simulink model "Electrical_System_2018b_obfs"  (R2019b)
settings: Solver=VariableStepAuto  StartTime=0.0  StopTime=5  RelTol=1e-3  AbsTol=1e-3  EnableMultiTasking=on
InitFcn:
  | Steady_State_Initialisation;
StopFcn:
  | %sscexplore(simlog);
  | %Logging
undefined symbols (not defined in the file): abrlhklxvp, aexgmhuedq, afmfmjnutg, afpphrjpnc, ahuxbyvruc, alarvljztt, amxnyqmnuw, aodrlwvqie, aolhmuplyq, aqpmguuqkg, auesgwirzl, aurophlnng, awamelrhru, ayfhvxflxn, azxkacuhqc, babszerikg, bawhdqanwq, bevoqecvei, bltjvqbchx, bmqsuewujl, bsmyqjfgnf, btvjbsmnve, bywgxqeadw, bziaduxaer, bzmcmdqocb, bzsvyvetat, ccsjnrbsih, cdvenygxwh, cedkrnslhx, cjheorclzs, cjrdshrtqx, ckhavyhcza, ckxewznhlz, cmrcgyiplk, conenicnws, cqkejbgjnn, csfnuwymhe, cunupkhwbh, cwzfvzuxxh, dcadmadufn, dcfponivnv, ddtrqjrhjn, dfhoxvkqas, dfrhtcwpne, dfvomcagjv, djijwylxea, dnmeqksrrm, dnzewbdkaa, dsqcykyxav, dtswwlttmm, ecumpidjtv, edegaywrct, ejjjsmnejc, eknqnehjdz, emvdetzouf, esxbqkbahr, etnkkbreiq, eunoiiiirw, ewewcuedir, fatkfxdhtc ... (+386)
libraries: fl_lib x802, ee_lib x362, fl_ps_legacy_lib x160, nesl_utility x85
(part 17 of 26)

== system Electrical_System_2018b_obfs/Redacted_1221/Redacted_7996/Redacted_7418/Redacted_4377/Redacted_6082/Redacted_1658 ==
  Redacted_1005 : fl_lib/Electrical/Electrical Elements/Switch  R_closed=ejlyeridsw Ohm  G_open=efsydslasd 1/Ohm  Threshold=qludltxvzj  i_specify=off  i_priority=None  i=qtqqggocjg A  i_nominal_specify=off  i_nominal_unit=A  i_nominal_value=irfgdwsyws  v_specify=off  v_priority=None  v=nrsfaplzum V  v_nominal_specify=off  v_nominal_unit=V  v_nominal_value=ffnnoojtnr
      settings: SourceProductName=Simscape
  Redacted_1354 : ee_lib/Passive/Thermal/Thermal Resistor  R=qdgpqkdjpo K/W  T_specify=off  T_priority=None  T=mtinxqvpod K  T_nominal_specify=off  T_nominal_unit=K  T_nominal_value=nyetipzdbd  Q_specify=off  Q_priority=None  Q=zeibppilau W  Q_nominal_specify=off  Q_nominal_unit=W  Q_nominal_value=ovthkmdajp
      settings: SourceProductName=Simscape Electrical  SourceProductBaseCode=PS  InternalSimscapePortConfiguration="{\"Bottom\":[],\"Left\":[{\"id\":\"A\",\"label\":\"A\",\"type\":\"foundation.thermal.thermal\"}],\"Right\":[{\"id\":\"B\",\"label\":\"B\",\"type\":\"foundation.thermal.thermal\"}],\"Top\":[]}"
  Redacted_3286 : ee_lib/Semiconductors & Converters/Diode  ModelType=qyiuharngl  Vf=uavesysmzd V  Ron=izxucsnofw Ohm  Goff=hxvsqjqvfr S  prmExp=jwlbdrgdyn  I12=fhtaelyvur A  V12=pntclgauty V  IS=xlgdpvdion A  ec=lsuwwyvoaz  I1=xioaihhcoe A  V1=prlupfwjwk V  RS=grfujeuioo Ohm  Tmeas=mmahtgxtlp degC  N_series=bdqkkbdoww  N_parallel=bdgudnfeam  Rz=vsyxoldpzj Ohm  BV=rczxpthhgf V  C_param=tlcavagjol  CJ=ssqnkrbywq pF  CJ0=wrromkkilg pF  VJ=faazhshxub V  Mgrad=ldrovslsoh  Vvec=vtbaecghrb V  Cvec=rijvdbsbjz pF  FC=ouvrtbvulr  Q_param=rrrehddltc  iRM=fyquguupcf A  iF=ikkfryheqp A  didt=scbuuymmti A/us  trr_factor=vwdzzjgtdl  trr=zktlrrknks ns  Qrr=utuviybabn s*uA  TT=jcgggencbc ns  tau=ssflxvsiut ns  T_param=nblvkicsaj  IS_T2=hpuqfgybtl A  I1_T2=atejcpbsmg A  V1_T2=txapzmzmbr V  Tmeas2=hogrcmodsn degC  EG_param=fwyzdxmfgf  EG=zfrilvllus eV  XTI_param=gxndnzccej  XTI=zngcdbbpek  dBVdT=ultmrnqodj V/K  Tdevice=cvuddcjgoa degC  i_specify=off  i_priority=None  i=xckzxtcuri A  i_nominal_specify=off  i_nominal_unit=A  i_nominal_value=mfjascwvwx  v_specify=off  v_priority=None  v=oytsestkkt V  v_nominal_specify=off  v_nominal_unit=V  v_nominal_value=rbtpehkrox  i_capacitor_specify=off  i_capacitor_priority=None  i_capacitor=lydrbpwfwm A  i_capacitor_nominal_specify=off  i_capacitor_nominal_unit=A  i_capacitor_nominal_value=gsonjyrsiu  v_capacitor_specify=off  v_capacitor_priority=None  v_capacitor=tlqtmxeebh V  v_capacitor_nominal_specify=off  v_capacitor_nominal_unit=V  v_capacitor_nominal_value=ixflknqnnv  power_dissipated_specify=off  power_dissipated_priority=None  power_dissipated=vhmskoronr W  power_dissipated_nominal_specify=off  power_dissipated_nominal_unit=W  power_dissipated_nominal_value=rqgtxqlwdp  thermal_network_parameterization=xkaopcnmoj  Rth=skumtgliel K/W  Rth_Foster=widqwnvljq K/W  thermal_mass_parameterization=ihdtigkqdr  thermal_mass=fxsrzmeque J/K  thermal_mass_Foster=cbmthsfafj J/K  thermal_time_constant=pmaqruvvqr s  thermal_time_constant_Foster=pxvwqyklyc s  thermal_mass_initial_temperatures=qerohrajht degC
      settings: SourceProductName=Simscape Electrical  InternalSimscapePortConfiguration="{\"Bottom\":[],\"Left\":[{\"id\":\"p\",\"label\":\"\",\"type\":\"foundation.electrical.electrical\"},{\"id\":\"H\",\"label\":\"H\",\"type\":\"foundation.thermal.thermal\"}],\"Right\":[{\"id\":\"n\",\"label\":\"\",\"type\":\"foundation.electrical.electrical\"}],\"Top\":[]}"
  Redacted_3861 : ee_lib/Semiconductors & Converters/Diode  ModelType=fxgsrmkiul  Vf=nwkiuphnod V  Ron=ytonkdenqd Ohm  Goff=vvxokjkhhi S  prmExp=rjijseurnu  I12=plnpdpppsb A  V12=clscpnwkyn V  IS=fgyrvtcpjw A  ec=myarsmgyax  I1=zaiuznwqub A  V1=urqjkvkqaz V  RS=atpbcqwqrk Ohm  Tmeas=avxaumhyvi degC  N_series=bdgfkyrlsu  N_parallel=cgmwatvtyk  Rz=jwremjkbfv Ohm  BV=kmqlppxuzg V  C_param=vvtbjwiqjw  CJ=dvukuyjagk pF  CJ0=ajovvjufex pF  VJ=lqxioxyjxp V  Mgrad=ugprrqpcng  Vvec=aycruakske V  Cvec=grqlqlzqyb pF  FC=xafzerxcin  Q_param=vnlbkyokpw  iRM=myuopxdhnp A  iF=wopzcdppvb A  didt=yoejpqomll A/us  trr_factor=vnzcsazbfp  trr=flnrjlmhdl ns  Qrr=abhmmrvgxl s*uA  TT=gfztyjvgqq ns  tau=oustnvpcaz ns  T_param=aznyhdnxgk  IS_T2=boxomshjpr A  I1_T2=imlgomczsp A  V1_T2=bhyftvbhbd V  Tmeas2=bhksuazwhb degC  EG_param=asaybnfknm  EG=gsrzwalape eV  XTI_param=duwkdllyki  XTI=aszcjfwkon  dBVdT=xhavbsykud V/K  Tdevice=nfydvwwomt degC  i_specify=off  i_priority=None  i=hibpeusmqj A  i_nominal_specify=off  i_nominal_unit=A  i_nominal_value=dgpnvsgdwn  v_specify=off  v_priority=None  v=xzghpqhkll V  v_nominal_specify=off  v_nominal_unit=V  v_nominal_value=aqwbnuvuma  i_capacitor_specify=off  i_capacitor_priority=None  i_capacitor=dbdawzejgx A  i_capacitor_nominal_specify=off  i_capacitor_nominal_unit=A  i_capacitor_nominal_value=skfhqqsyjv  v_capacitor_specify=off  v_capacitor_priority=None  v_capacitor=kngohrnxjb V  v_capacitor_nominal_specify=off  v_capacitor_nominal_unit=V  v_capacitor_nominal_value=knpvixzgdi  power_dissipated_specify=off  power_dissipated_priority=None  power_dissipated=zhfsmmbryx W  power_dissipated_nominal_specify=off  power_dissipated_nominal_unit=W  power_dissipated_nominal_value=oxbqwsyfdo  thermal_network_parameterization=gluxlhswsh  Rth=wkzzkloygz K/W  Rth_Foster=lchzecrkjz K/W  thermal_mass_parameterization=gwvmgktbjo  thermal_mass=rmhlykpfbd J/K  thermal_mass_Foster=ahdrbmndbt J/K  thermal_time_constant=geccsojpnx s  thermal_time_constant_Foster=oeduphnpru s  thermal_mass_initial_temperatures=wnupirfodr degC
      settings: SourceProductName=Simscape Electrical  InternalSimscapePortConfiguration="{\"Bottom\":[],\"Left\":[{\"id\":\"p\",\"label\":\"\",\"type\":\"foundation.electrical.electrical\"},{\"id\":\"H\",\"label\":\"H\",\"type\":\"foundation.thermal.thermal\"}],\"Right\":[{\"id\":\"n\",\"label\":\"\",\"type\":\"foundation.electrical.electrical\"}],\"Top\":[]}"
  Redacted_5977 : fl_lib/Electrical/Electrical Elements/Switch  R_closed=cjwmmdrupk Ohm  G_open=qstxdugiyk 1/Ohm  Threshold=kztcpnpmvs  i_specify=off  i_priority=None  i=lmxbtdndwg A  i_nominal_specify=off  i_nominal_unit=A  i_nominal_value=qyeufjvfiw  v_specify=off  v_priority=None  v=gastazzonl V  v_nominal_specify=off  v_nominal_unit=V  v_nominal_value=mjiwwishzy
      settings: SourceProductName=Simscape
  Redacted_6041 : ee_lib/Passive/Thermal/Thermal Resistor  R=xbcnqysxek K/W  T_specify=off  T_priority=None  T=bzsvyvetat K  T_nominal_specify=off  T_nominal_unit=K  T_nominal_value=ewqiuajrkb  Q_specify=off  Q_priority=None  Q=jhzrvwpmgk W  Q_nominal_specify=off  Q_nominal_unit=W  Q_nominal_value=tohlmuixqc
      settings: SourceProductName=Simscape Electrical  SourceProductBaseCode=PS  InternalSimscapePortConfiguration="{\"Bottom\":[],\"Left\":[{\"id\":\"A\",\"label\":\"A\",\"type\":\"foundation.thermal.thermal\"}],\"Right\":[{\"id\":\"B\",\"label\":\"B\",\"type\":\"foundation.thermal.thermal\"}],\"Top\":[]}"
  Redacted_7612 : ee_lib/Passive/Thermal/Thermal Resistor  R=ogtgsqkykv K/W  T_specify=off  T_priority=None  T=welbpoxbdd K  T_nominal_specify=off  T_nominal_unit=K  T_nominal_value=owcjlhxdxh  Q_specify=off  Q_priority=None  Q=jawtmfuqev W  Q_nominal_specify=off  Q_nominal_unit=W  Q_nominal_value=amvswbkqpm
      settings: SourceProductName=Simscape Electrical  SourceProductBaseCode=PS  InternalSimscapePortConfiguration="{\"Bottom\":[],\"Left\":[{\"id\":\"A\",\"label\":\"A\",\"type\":\"foundation.thermal.thermal\"}],\"Right\":[{\"id\":\"B\",\"label\":\"B\",\"type\":\"foundation.thermal.thermal\"}],\"Top\":[]}"
  Redacted_4312 : PMIOPort  Side=Left
  Redacted_7440 : PMIOPort  Port=2  Side=Left
  Redacted_7574 : PMIOPort  Port=3  Side=Right
  Redacted_5998 : PMIOPort  Port=4  Side=Right
  Redacted_5346 : PMIOPort  Port=5  Side=Left
  Redacted_698 : PMIOPort  Port=6  Side=Right
  connections:
  Redacted_3861/LConn2 -- Redacted_7612/LConn1
  Redacted_6041/RConn1 -- Redacted_5346/RConn1
  Redacted_5998/RConn1 -- Redacted_5977/RConn2
  Redacted_1005/RConn1 -- Redacted_5977/RConn1 -- Redacted_698/RConn1
  Redacted_1354/RConn1 -- Redacted_6041/LConn1 -- Redacted_7612/RConn1
  Redacted_4312/RConn1 -- Redacted_3286/RConn1
  Redacted_3286/LConn1 -- Redacted_1005/LConn1
  Redacted_7574/RConn1 -- Redacted_1005/RConn2
  Redacted_3286/LConn2 -- Redacted_1354/LConn1
  Redacted_3861/RConn1 -- Redacted_5977/LConn1
  Redacted_3861/LConn1 -- Redacted_7440/RConn1

== system Electrical_System_2018b_obfs/Redacted_1221/Redacted_7996/Redacted_7418/Redacted_4377/Redacted_6082/Redacted_1843 ==
  Neutral_Negative : Subsystem  VariantControl=Variant1
  Positive_Neutral : Subsystem  VariantControl=Variant3
  Redacted_8971 : Subsystem  VariantControl=Variant2
  Redacted_2601 : PMIOPort  Side=Left
  Redacted_5367 : PMIOPort  Port=2  Side=Left
  Redacted_1109 : PMIOPort  Port=3  Side=Left
  Redacted_4235 : PMIOPort  Port=4  Side=Right
  Redacted_9086 : PMIOPort  Port=5  Side=Right

== system Electrical_System_2018b_obfs/Redacted_1221/Redacted_7996/Redacted_7418/Redacted_4377/Redacted_6082/Redacted_1901 ==
  Redacted_1229 : ee_lib/Passive/Thermal/Thermal Resistor  R=hfneeleggr K/W  T_specify=off  T_priority=None  T=dnmeqksrrm K  T_nominal_specify=off  T_nominal_unit=K  T_nominal_value=uhclxpopbh  Q_specify=off  Q_priority=None  Q=nyzppyukeu W  Q_nominal_specify=off  Q_nominal_unit=W  Q_nominal_value=mrympoiojz
      settings: SourceProductName=Simscape Electrical  SourceProductBaseCode=PS  InternalSimscapePortConfiguration="{\"Bottom\":[],\"Left\":[{\"id\":\"A\",\"label\":\"A\",\"type\":\"foundation.thermal.thermal\"}],\"Right\":[{\"id\":\"B\",\"label\":\"B\",\"type\":\"foundation.thermal.thermal\"}],\"Top\":[]}"
  Redacted_1317 : ee_lib/Passive/Thermal/Thermal Resistor  R=ddtrqjrhjn K/W  T_specify=off  T_priority=None  T=myvnfneauu K  T_nominal_specify=off  T_nominal_unit=K  T_nominal_value=vndthaumwj  Q_specify=off  Q_priority=None  Q=jvrrmptdue W  Q_nominal_specify=off  Q_nominal_unit=W  Q_nominal_value=zyzovxzrox
      settings: SourceProductName=Simscape Electrical  SourceProductBaseCode=PS  InternalSimscapePortConfiguration="{\"Bottom\":[],\"Left\":[{\"id\":\"A\",\"label\":\"A\",\"type\":\"foundation.thermal.thermal\"}],\"Right\":[{\"id\":\"B\",\"label\":\"B\",\"type\":\"foundation.thermal.thermal\"}],\"Top\":[]}"
  Redacted_2918 : ee_lib/Semiconductors & Converters/Diode  ModelType=tboxenabfk  Vf=ysocghjvnj V  Ron=igyyqbbazt Ohm  Goff=wrcmatehqh S  prmExp=umofwxphaz  I12=boewnunols A  V12=agfxygazzy V  IS=yxpwlphqya A  ec=ezskytlukg  I1=hfmdeevxjm A  V1=lbjfenfgli V  RS=crmaftxtdn Ohm  Tmeas=rzhxrfhrws degC  N_series=qhotvmyapg  N_parallel=dcamtsthwp  Rz=qwnnbscosu Ohm  BV=bgsuezylxr V  C_param=jefhggiqkq  CJ=nrftpgzbwn pF  CJ0=vpkmzxlujx pF  VJ=nqopqysaak V  Mgrad=jnpgifqefs  Vvec=cniqwxpvbi V  Cvec=plwpepcsqe pF  FC=gzewllqrkw  Q_param=xlnrldobms  iRM=ytqzliqbll A  iF=svsqnejsfr A  didt=lrnrbryckm A/us  trr_factor=qpcgqhjpel  trr=emvijkzjdz ns  Qrr=ykzfmghaqw s*uA  TT=cegrsucons ns  tau=hhbhhwwsxm ns  T_param=jxhekmoycn  IS_T2=cnunlqxwqa A  I1_T2=tqdiqvzzvb A  V1_T2=ukgedxicts V  Tmeas2=ypzgidmcky degC  EG_param=ahptxqtjkj  EG=pprjzflisz eV  XTI_param=luwukgfqqn  XTI=bnvhtyteod  dBVdT=loswkuonel V/K  Tdevice=ctewjlisga degC  i_specify=off  i_priority=None  i=kufuhybcxo A  i_nominal_specify=off  i_nominal_unit=A  i_nominal_value=fnodmzekrv  v_specify=off  v_priority=None  v=bvjjoninjh V  v_nominal_specify=off  v_nominal_unit=V  v_nominal_value=wmrqkzdvam  i_capacitor_specify=off  i_capacitor_priority=None  i_capacitor=sawezjxpgh A  i_capacitor_nominal_specify=off  i_capacitor_nominal_unit=A  i_capacitor_nominal_value=dzrakfqruq  v_capacitor_specify=off  v_capacitor_priority=None  v_capacitor=ckefveljbv V  v_capacitor_nominal_specify=off  v_capacitor_nominal_unit=V  v_capacitor_nominal_value=zlbmprnqfe  power_dissipated_specify=off  power_dissipated_priority=None  power_dissipated=npelzyxkbr W  power_dissipated_nominal_specify=off  power_dissipated_nominal_unit=W  power_dissipated_nominal_value=xyqqsiyxsx  thermal_network_parameterization=cmpqaimztb  Rth=fyfjdoegdn K/W  Rth_Foster=ouazsjqzqc K/W  thermal_mass_parameterization=uskugrezwe  thermal_mass=kfppvbxohl J/K  thermal_mass_Foster=iohubghcog J/K  thermal_time_constant=tbegstwujr s  thermal_time_constant_Foster=kbaqkpxwop s  thermal_mass_initial_temperatures=tmxmgoawom degC
      settings: SourceProductName=Simscape Electrical  InternalSimscapePortConfiguration="{\"Bottom\":[],\"Left\":[{\"id\":\"p\",\"label\":\"\",\"type\":\"foundation.electrical.electrical\"},{\"id\":\"H\",\"label\":\"H\",\"type\":\"foundation.thermal.thermal\"}],\"Right\":[{\"id\":\"n\",\"label\":\"\",\"type\":\"foundation.electrical.electrical\"}],\"Top\":[]}"
  Redacted_3887 : ee_lib/Semiconductors & Converters/Diode  ModelType=kgpqvwzuvf  Vf=pusmgjlfhw V  Ron=zdvhkofkio Ohm  Goff=rrsomwrhky S  prmExp=puvexjufpm  I12=tlbhkktqov A  V12=jgzzzcxugv V  IS=pqeeblyemi A  ec=yagdawcefa  I1=baiumjodsv A  V1=kvrziecayr V  RS=emddjdnqya Ohm  Tmeas=kukopsdiuw degC  N_series=rabuyhqlar  N_parallel=fzdlculjid  Rz=oyqbhoxixc Ohm  BV=powcerqowi V  C_param=aeoqkmsqgo  CJ=omumwwbzoq pF  CJ0=sznaxolwxw pF  VJ=kdgpnhjdki V  Mgrad=owoxwkiptx  Vvec=yphehuqnex V  Cvec=yioiudmgas pF  FC=diwfpfnlom  Q_param=cswgmtympe  iRM=nsikknuycn A  iF=udnoipznau A  didt=omhhheqqis A/us  trr_factor=kiajvubcqx  trr=eifapbzssj ns  Qrr=igpekaohrl s*uA  TT=jucdrpilud ns  tau=lahsbpxgyi ns  T_param=vnthpegzri  IS_T2=edtnoyclnw A  I1_T2=emvajrspsy A  V1_T2=nghezzebkw V  Tmeas2=etfqwqeleu degC  EG_param=fmhucqmugz  EG=ytvyyycxld eV  XTI_param=kxpyactpjk  XTI=ijcctumawz  dBVdT=mveoqdoxea V/K  Tdevice=rasndouawu degC  i_specify=off  i_priority=None  i=middmtxema A  i_nominal_specify=off  i_nominal_unit=A  i_nominal_value=ulcnzrhotg  v_specify=off  v_priority=None  v=cirgoxespi V  v_nominal_specify=off  v_nominal_unit=V  v_nominal_value=dnkswukuqy  i_capacitor_specify=off  i_capacitor_priority=None  i_capacitor=uvmqwudjqx A  i_capacitor_nominal_specify=off  i_capacitor_nominal_unit=A  i_capacitor_nominal_value=tjhsaljlzi  v_capacitor_specify=off  v_capacitor_priority=None  v_capacitor=gtauwsvkmg V  v_capacitor_nominal_specify=off  v_capacitor_nominal_unit=V  v_capacitor_nominal_value=yrtxkgmrjc  power_dissipated_specify=off  power_dissipated_priority=None  power_dissipated=gejrmthogs W  power_dissipated_nominal_specify=off  power_dissipated_nominal_unit=W  power_dissipated_nominal_value=fnkdipvfax  thermal_network_parameterization=brstcitzoq  Rth=qauyoickxf K/W  Rth_Foster=pcmfvqnjph K/W  thermal_mass_parameterization=csstahwskj  thermal_mass=uinbpeizom J/K  thermal_mass_Foster=udgsofajzw J/K  thermal_time_constant=fbszgisaxv s  thermal_time_constant_Foster=qzpyvzuxkn s  thermal_mass_initial_temperatures=tcrrrnbkcb degC
      settings: SourceProductName=Simscape Electrical  InternalSimscapePortConfiguration="{\"Bottom\":[],\"Left\":[{\"id\":\"p\",\"label\":\"\",\"type\":\"foundation.electrical.electrical\"},{\"id\":\"H\",\"label\":\"H\",\"type\":\"foundation.thermal.thermal\"}],\"Right\":[{\"id\":\"n\",\"label\":\"\",\"type\":\"foundation.electrical.electrical\"}],\"Top\":[]}"
  Redacted_5062 : fl_lib/Electrical/Electrical Elements/Switch  R_closed=ajgjjzldor Ohm  G_open=aanuvbeift 1/Ohm  Threshold=fyvpcwnmem  i_specify=off  i_priority=None  i=farnwkyrka A  i_nominal_specify=off  i_nominal_unit=A  i_nominal_value=uzlteuglkb  v_specify=off  v_priority=None  v=tekycmpguo V  v_nominal_specify=off  v_nominal_unit=V  v_nominal_value=hyrhbabztl
      settings: SourceProductName=Simscape
  Redacted_6145 : fl_lib/Electrical/Electrical Elements/Switch  R_closed=wzxtffzhqk Ohm  G_open=ttmifnbefi 1/Ohm  Threshold=zzdsjwvyov  i_specify=off  i_priority=None  i=wibaukydmt A  i_nominal_specify=off  i_nominal_unit=A  i_nominal_value=shaiddzzkm  v_specify=off  v_priority=None  v=adhjlkibew V  v_nominal_specify=off  v_nominal_unit=V  v_nominal_value=ctlxurrbzu
      settings: SourceProductName=Simscape
  Redacted_8303 : ee_lib/Passive/Thermal/Thermal Resistor  R=dcadmadufn K/W  T_specify=off  T_priority=None  T=kapvbwdbts K  T_nominal_specify=off  T_nominal_unit=K  T_nominal_value=ghgowxtkgp  Q_specify=off  Q_priority=None  Q=amzvaiirbc W  Q_nominal_specify=off  Q_nominal_unit=W  Q_nominal_value=ptxjogujxs
      settings: SourceProductName=Simscape Electrical  SourceProductBaseCode=PS  InternalSimscapePortConfiguration="{\"Bottom\":[],\"Left\":[{\"id\":\"A\",\"label\":\"A\",\"type\":\"foundation.thermal.thermal\"}],\"Right\":[{\"id\":\"B\",\"label\":\"B\",\"type\":\"foundation.thermal.thermal\"}],\"Top\":[]}"
  Redacted_8116 : PMIOPort  Side=Left
  Redacted_9290 : PMIOPort  Port=2  Side=Left
  Redacted_6411 : PMIOPort  Port=3  Side=Right
  Redacted_9481 : PMIOPort  Port=4  Side=Right
  Redacted_1243 : PMIOPort  Port=5  Side=Left
  Redacted_5181 : PMIOPort  Port=6  Side=Right
  connections:
  Redacted_3887/LConn1 -- Redacted_9290/RConn1
  Redacted_3887/RConn1 -- Redacted_6145/LConn1
  Redacted_2918/LConn2 -- Redacted_1229/LConn1
  Redacted_6411/RConn1 -- Redacted_5062/RConn2
  Redacted_2918/LConn1 -- Redacted_5062/LConn1
  Redacted_8116/RConn1 -- Redacted_2918/RConn1
  Redacted_1317/RConn1 -- Redacted_8303/LConn1 -- Redacted_1229/RConn1
  Redacted_5181/RConn1 -- Redacted_6145/RConn1 -- Redacted_5062/RConn1
  Redacted_9481/RConn1 -- Redacted_6145/RConn2
  Redacted_8303/RConn1 -- Redacted_1243/RConn1
  Redacted_3887/LConn2 -- Redacted_1317/LConn1

== system Electrical_System_2018b_obfs/Redacted_1221/Redacted_7996/Redacted_7418/Redacted_4377/Redacted_6082/Redacted_2005 ==
  Neutral_Negative : Subsystem  VariantControl=Variant1
  Positive_Neutral : Subsystem  VariantControl=Variant3
  Redacted_335 : Subsystem  VariantControl=Variant2
  Redacted_8266 : PMIOPort  Side=Left
  Redacted_1423 : PMIOPort  Port=2  Side=Left
  Redacted_7633 : PMIOPort  Port=3  Side=Left
  Redacted_8552 : PMIOPort  Port=4  Side=Right
  Redacted_2441 : PMIOPort  Port=5  Side=Right

== system Electrical_System_2018b_obfs/Redacted_1221/Redacted_7996/Redacted_7418/Redacted_4377/Redacted_6082/Redacted_2122 ==
  Neutral_Negative : Subsystem  VariantControl=Variant1
  Positive_Neutral : Subsystem  VariantControl=Variant3
  Redacted_1391 : Subsystem  VariantControl=Variant2
  Redacted_659 : PMIOPort  Side=Left
  Redacted_1619 : PMIOPort  Port=2  Side=Left
  Redacted_5171 : PMIOPort  Port=3  Side=Left
  Redacted_2219 : PMIOPort  Port=4  Side=Right
  Redacted_5591 : PMIOPort  Port=5  Side=Right

== system Electrical_System_2018b_obfs/Redacted_1221/Redacted_7996/Redacted_7418/Redacted_4377/Redacted_6082/Redacted_2183 ==
  Redacted_1396 : fl_lib/Electrical/Electrical Elements/Switch  R_closed=wmcpxqyfeh Ohm  G_open=ordboroxst 1/Ohm  Threshold=puyanqdwrl  i_specify=off  i_priority=None  i=bnajmanprt A  i_nominal_specify=off  i_nominal_unit=A  i_nominal_value=rlbcudmlql  v_specify=off  v_priority=None  v=cqbyhwtmeu V  v_nominal_specify=off  v_nominal_unit=V  v_nominal_value=ssehunbzon
      settings: SourceProductName=Simscape
  Redacted_3366 : ee_lib/Passive/Thermal/Thermal Resistor  R=bawhdqanwq K/W  T_specify=off  T_priority=None  T=nptyawlpaq K  T_nominal_specify=off  T_nominal_unit=K  T_nominal_value=finlbxanjw  Q_specify=off  Q_priority=None  Q=alilpavgri W  Q_nominal_specify=off  Q_nominal_unit=W  Q_nominal_value=wneqapuicx
      settings: SourceProductName=Simscape Electrical  SourceProductBaseCode=PS  InternalSimscapePortConfiguration="{\"Bottom\":[],\"Left\":[{\"id\":\"A\",\"label\":\"A\",\"type\":\"foundation.thermal.thermal\"}],\"Right\":[{\"id\":\"B\",\"label\":\"B\",\"type\":\"foundation.thermal.thermal\"}],\"Top\":[]}"
  Redacted_4085 : fl_lib/Electrical/Electrical Elements/Switch  R_closed=jdqhtjuyba Ohm  G_open=nqhnggplew 1/Ohm  Threshold=jecqzekwwf  i_specify=off  i_priority=None  i=parwtazsiw A  i_nominal_specify=off  i_nominal_unit=A  i_nominal_value=cbscxuyyvd  v_specify=off  v_priority=None  v=prtofmgyxi V  v_nominal_specify=off  v_nominal_unit=V  v_nominal_value=ygccoktkvx
      settings: SourceProductName=Simscape
  Redacted_6327 : ee_lib/Semiconductors & Converters/Diode  ModelType=wmwpyziqse  Vf=hsrvymleww V  Ron=pyrhpbxgop Ohm  Goff=ooooykpefi S  prmExp=fgnltfxrhl  I12=dbygefiygg A  V12=yxnireldoj V  IS=umytqsawsi A  ec=rwknegxugi  I1=qflroumpgm A  V1=riphrjudsb V  RS=tsfshgyhqz Ohm  Tmeas=qkexvrxdoi degC  N_series=cbszsjtyip  N_parallel=ybgzghthgk  Rz=gkwnarnzwz Ohm  BV=yqgteuoupv V  C_param=taxfohzknz  CJ=lmergqmyrh pF  CJ0=qfikrlcnko pF  VJ=zrhpkoalsk V  Mgrad=ztoncwtqia  Vvec=lyykpwvhzi V  Cvec=gasstcbauf pF  FC=eeghpxvwex  Q_param=fnbxqtfxwi  iRM=zmetzqvpxi A  iF=tsqxkbkjzp A  didt=celvxerdut A/us  trr_factor=ciexehbuux  trr=pmnqwrbgch ns  Qrr=rvaiuqfkvk s*uA  TT=lwokilfxpw ns  tau=ydjtzutwsj ns  T_param=rezrybflyz  IS_T2=whhobjfmpx A  I1_T2=fbtorsgebe A  V1_T2=lcyuerboic V  Tmeas2=ffdvqttstk degC  EG_param=qyhjbidgce  EG=sjwyndroxb eV  XTI_param=sliofzfaaf  XTI=sksaqpzvmm  dBVdT=zooqrpscpn V/K  Tdevice=docgwdkzmk degC  i_specify=off  i_priority=None  i=rmpavrhrmg A  i_nominal_specify=off  i_nominal_unit=A  i_nominal_value=sblhgjjhtn  v_specify=off  v_priority=None  v=tqvxxaryfu V  v_nominal_specify=off  v_nominal_unit=V  v_nominal_value=zbwqzplush  i_capacitor_specify=off  i_capacitor_priority=None  i_capacitor=ozsqayjyjj A  i_capacitor_nominal_specify=off  i_capacitor_nominal_unit=A  i_capacitor_nominal_value=bwqctegvbe  v_capacitor_specify=off  v_capacitor_priority=None  v_capacitor=msafonbusr V  v_capacitor_nominal_specify=off  v_capacitor_nominal_unit=V  v_capacitor_nominal_value=alqpnbtqbu  power_dissipated_specify=off  power_dissipated_priority=None  power_dissipated=ldpizezrgb W  power_dissipated_nominal_specify=off  power_dissipated_nominal_unit=W  power_dissipated_nominal_value=jdcvhdvcqn  thermal_network_parameterization=khqyflkkbo  Rth=hbtoumkpux K/W  Rth_Foster=owtwhhuqef K/W  thermal_mass_parameterization=tyagarpfgc  thermal_mass=odjqiqbmnv J/K  thermal_mass_Foster=dpqmogzzyw J/K  thermal_time_constant=nrygysvakb s  thermal_time_constant_Foster=pknwccaesz s  thermal_mass_initial_temperatures=ubqttyiytq degC
      settings: SourceProductName=Simscape Electrical  InternalSimscapePortConfiguration="{\"Bottom\":[],\"Left\":[{\"id\":\"p\",\"label\":\"\",\"type\":\"foundation.electrical.electrical\"},{\"id\":\"H\",\"label\":\"H\",\"type\":\"foundation.thermal.thermal\"}],\"Right\":[{\"id\":\"n\",\"label\":\"\",\"type\":\"foundation.electrical.electrical\"}],\"Top\":[]}"
  Redacted_6920 : ee_lib/Semiconductors & Converters/Diode  ModelType=ifkeajuogy  Vf=rvxoqojvbw V  Ron=wlhpwjfqxp Ohm  Goff=bvtpgzsrrx S  prmExp=nlergzwjbu  I12=cxqwsuomth A  V12=vmavhsfifk V  IS=eyymhspphz A  ec=yiafetqxro  I1=hmubrgwopc A  V1=lmsucbmfuc V  RS=ebxfexknak Ohm  Tmeas=pmaoxtpzfm degC  N_series=kbcwisxpjg  N_parallel=aaklmjotsd  Rz=pkzujcjpob Ohm  BV=gdhqaesgrk V  C_param=qtgcbvllfp  CJ=qsggiorgze pF  CJ0=sddrldehqk pF  VJ=ednypbqmsy V  Mgrad=ynapqanrdu  Vvec=zhnqfijbdq V  Cvec=brtmpahjnt pF  FC=znsqocjczl  Q_param=aczsqxqrku  iRM=kkzlynschx A  iF=weflpmxsur A  didt=ifitwlscxo A/us  trr_factor=cwbxopwcbm  trr=ozwjbkszwz ns  Qrr=tosvjxaqxp s*uA  TT=vwmcrpsobc ns  tau=yavnmcqbxl ns  T_param=bfahnjcmju  IS_T2=iahumvdhta A  I1_T2=omfubwbwfi A  V1_T2=adpnfnmwdl V  Tmeas2=vfowspfngr degC  EG_param=qfnvybezbd  EG=pzpugzngnq eV  XTI_param=acwvpdokxd  XTI=tmjvpeiptd  dBVdT=yiwxmdmzvv V/K  Tdevice=mpkhxzqybm degC  i_specify=off  i_priority=None  i=zsqooaqzpu A  i_nominal_specify=off  i_nominal_unit=A  i_nominal_value=trowwbswpb  v_specify=off  v_priority=None  v=buogftaazb V  v_nominal_specify=off  v_nominal_unit=V  v_nominal_value=qjdjlsbbbw  i_capacitor_specify=off  i_capacitor_priority=None  i_capacitor=siqvzgfjbj A  i_capacitor_nominal_specify=off  i_capacitor_nominal_unit=A  i_capacitor_nominal_value=jygxpnflsn  v_capacitor_specify=off  v_capacitor_priority=None  v_capacitor=auwydfvsni V  v_capacitor_nominal_specify=off  v_capacitor_nominal_unit=V  v_capacitor_nominal_value=ouyytgmkij  power_dissipated_specify=off  power_dissipated_priority=None  power_dissipated=hyulojmtmo W  power_dissipated_nominal_specify=off  power_dissipated_nominal_unit=W  power_dissipated_nominal_value=qbvoqhgkhp  thermal_network_parameterization=ppykqmtlhl  Rth=glausydyft K/W  Rth_Foster=fkytfeohhw K/W  thermal_mass_parameterization=oluvrdypml  thermal_mass=fnhzvqgtxn J/K  thermal_mass_Foster=ppzvcmktwx J/K  thermal_time_constant=dhlpwbmywt s  thermal_time_constant_Foster=gidfxyibkk s  thermal_mass_initial_temperatures=korqzmgtir degC
      settings: SourceProductName=Simscape Electrical  InternalSimscapePortConfiguration="{\"Bottom\":[],\"Left\":[{\"id\":\"p\",\"label\":\"\",\"type\":\"foundation.electrical.electrical\"},{\"id\":\"H\",\"label\":\"H\",\"type\":\"foundation.thermal.thermal\"}],\"Right\":[{\"id\":\"n\",\"label\":\"\",\"type\":\"foundation.electrical.electrical\"}],\"Top\":[]}"
  Redacted_8780 : ee_lib/Passive/Thermal/Thermal Resistor  R=lykhbhfuku K/W  T_specify=off  T_priority=None  T=qujobzntab K  T_nominal_specify=off  T_nominal_unit=K  T_nominal_value=fwjjrigoji  Q_specify=off  Q_priority=None  Q=oyodymkfqm W  Q_nominal_specify=off  Q_nominal_unit=W  Q_nominal_value=ecbnragssr
      settings: SourceProductName=Simscape Electrical  SourceProductBaseCode=PS  InternalSimscapePortConfiguration="{\"Bottom\":[],\"Left\":[{\"id\":\"A\",\"label\":\"A\",\"type\":\"foundation.thermal.thermal\"}],\"Right\":[{\"id\":\"B\",\"label\":\"B\",\"type\":\"foundation.thermal.thermal\"}],\"Top\":[]}"
  Redacted_8981 : ee_lib/Passive/Thermal/Thermal Resistor  R=gcimydvvyd K/W  T_specify=off  T_priority=None  T=seiwuzyrmn K  T_nominal_specify=off  T_nominal_unit=K  T_nominal_value=nxsogkjqln  Q_specify=off  Q_priority=None  Q=iroscqsegj W  Q_nominal_specify=off  Q_nominal_unit=W  Q_nominal_value=bqfmelgyip
      settings: SourceProductName=Simscape Electrical  SourceProductBaseCode=PS  InternalSimscapePortConfiguration="{\"Bottom\":[],\"Left\":[{\"id\":\"A\",\"label\":\"A\",\"type\":\"foundation.thermal.thermal\"}],\"Right\":[{\"id\":\"B\",\"label\":\"B\",\"type\":\"foundation.thermal.thermal\"}],\"Top\":[]}"
  Redacted_9228 : PMIOPort  Side=Left
  Redacted_927 : PMIOPort  Port=2  Side=Left
  Redacted_1010 : PMIOPort  Port=3  Side=Right
  Redacted_500 : PMIOPort  Port=4  Side=Right
  Redacted_1718 : PMIOPort  Port=5  Side=Left
  Redacted_7712 : PMIOPort  Port=6  Side=Right
  connections:
  Redacted_6920/LConn2 -- Redacted_3366/LConn1
  Redacted_8981/RConn1 -- Redacted_1718/RConn1
  Redacted_500/RConn1 -- Redacted_1396/RConn2
  Redacted_4085/RConn1 -- Redacted_1396/RConn1 -- Redacted_7712/RConn1
  Redacted_8780/RConn1 -- Redacted_8981/LConn1 -- Redacted_3366/RConn1
  Redacted_9228/RConn1 -- Redacted_6327/RConn1
  Redacted_6327/LConn1 -- Redacted_4085/LConn1
  Redacted_1010/RConn1 -- Redacted_4085/RConn2
  Redacted_6327/LConn2 -- Redacted_8780/LConn1
  Redacted_6920/RConn1 -- Redacted_1396/LConn1
  Redacted_6920/LConn1 -- Redacted_927/RConn1

== system Electrical_System_2018b_obfs/Redacted_1221/Redacted_7996/Redacted_7418/Redacted_4377/Redacted_6082/Redacted_2443 ==
  Neutral_Negative : Subsystem  VariantControl=Variant1
  Positive_Neutral : Subsystem  VariantControl=Variant3
  Redacted_6791 : Subsystem  VariantControl=Variant2
  Redacted_2078 : PMIOPort  Side=Left
  Redacted_827 : PMIOPort  Port=2  Side=Left
  Redacted_65 : PMIOPort  Port=3  Side=Left
  Redacted_2555 : PMIOPort  Port=4  Side=Right
  Redacted_7416 : PMIOPort  Port=5  Side=Right

== system Electrical_System_2018b_obfs/Redacted_1221/Redacted_7996/Redacted_7418/Redacted_4377/Redacted_6082/Redacted_248 ==
  Neutral_Negative : Subsystem  VariantControl=Variant1
  Positive_Neutral : Subsystem  VariantControl=Variant3
  Redacted_2281 : Subsystem  VariantControl=Variant2
  Redacted_4518 : PMIOPort  Side=Left
  Redacted_7536 : PMIOPort  Port=2  Side=Left
  Redacted_9561 : PMIOPort  Port=3  Side=Left
  Redacted_1518 : PMIOPort  Port=4  Side=Right
  Redacted_7660 : PMIOPort  Port=5  Side=Right

== system Electrical_System_2018b_obfs/Redacted_1221/Redacted_7996/Redacted_7418/Redacted_4377/Redacted_6082/Redacted_2710 ==
  Redacted_1835 : ee_lib/Passive/Thermal/Thermal Resistor  R=zuzrchwspe K/W  T_specify=off  T_priority=None  T=eunoiiiirw K  T_nominal_specify=off  T_nominal_unit=K  T_nominal_value=yftlbkraoc  Q_specify=off  Q_priority=None  Q=kaqhtzlkmw W  Q_nominal_specify=off  Q_nominal_unit=W  Q_nominal_value=kxsmqmphud
      settings: SourceProductName=Simscape Electrical  SourceProductBaseCode=PS  InternalSimscapePortConfiguration="{\"Bottom\":[],\"Left\":[{\"id\":\"A\",\"label\":\"A\",\"type\":\"foundation.thermal.thermal\"}],\"Right\":[{\"id\":\"B\",\"label\":\"B\",\"type\":\"foundation.thermal.thermal\"}],\"Top\":[]}"
  Redacted_2325 : ee_lib/Passive/Thermal/Thermal Resistor  R=oohwiocpwa K/W  T_specify=off  T_priority=None  T=aodrlwvqie K  T_nominal_specify=off  T_nominal_unit=K  T_nominal_value=hbqkshwgbe  Q_specify=off  Q_priority=None  Q=zgbdrenlos W  Q_nominal_specify=off  Q_nominal_unit=W  Q_nominal_value=gyllwstqdw
      settings: SourceProductName=Simscape Electrical  SourceProductBaseCode=PS  InternalSimscapePortConfiguration="{\"Bottom\":[],\"Left\":[{\"id\":\"A\",\"label\":\"A\",\"type\":\"foundation.thermal.thermal\"}],\"Right\":[{\"id\":\"B\",\"label\":\"B\",\"type\":\"foundation.thermal.thermal\"}],\"Top\":[]}"
  Redacted_24 : ee_lib/Semiconductors & Converters/Diode  ModelType=divufniqhz  Vf=fuswyfzioa V  Ron=sfkcggclsz Ohm  Goff=rpmhprrivu S  prmExp=rqsfzusaiw  I12=cqrlsxwtvu A  V12=gimzrykmwg V  IS=rbknwvhbll A  ec=ygxdpgkrus  I1=tarfhsbhda A  V1=auwltsmvvt V  RS=troyncdmko Ohm  Tmeas=dpmoufhgnq degC  N_series=mqgkycpjnt  N_parallel=iatvhhkcmg  Rz=fwzkufafef Ohm  BV=zmpddawwjp V  C_param=qikpakizwp  CJ=hljtvaqupa pF  CJ0=oewuaitods pF  VJ=xrrquippxs V  Mgrad=oyxruwepxk  Vvec=iunesjqkcl V  Cvec=vvxzfuxhsc pF  FC=wwyulevwwe  Q_param=sttqtkaprf  iRM=ykusalgnes A  iF=pvzoejfzxx A  didt=adheigkzej A/us  trr_factor=oeawnjlela  trr=nbebmwvdrw ns  Qrr=lgxgfdaswr s*uA  TT=mupppamadl ns  tau=pradyztspj ns  T_param=djosuqmtzl  IS_T2=kouzrlehuq A  I1_T2=ovjcqjjnvt A  V1_T2=fvujieyhhk V  Tmeas2=epvpjdnelz degC  EG_param=qptvtngyyt  EG=ndvbbapzev eV  XTI_param=msvaynwzcp  XTI=cmxevtkdww  dBVdT=pyfqnygnab V/K  Tdevice=rmrhsufjav degC  i_specify=off  i_priority=None  i=wbjfwxwcps A  i_nominal_specify=off  i_nominal_unit=A  i_nominal_value=npkrcglwju  v_specify=off  v_priority=None  v=pdjfweujkd V  v_nominal_specify=off  v_nominal_unit=V  v_nominal_value=ipmoxmdjvx  i_capacitor_specify=off  i_capacitor_priority=None  i_capacitor=tlbvdlttjz A  i_capacitor_nominal_specify=off  i_capacitor_nominal_unit=A  i_capacitor_nominal_value=lexosykyas  v_capacitor_specify=off  v_capacitor_priority=None  v_capacitor=tjzvbhzdbm V  v_capacitor_nominal_specify=off  v_capacitor_nominal_unit=V  v_capacitor_nominal_value=bewlyffcpp  power_dissipated_specify=off  power_dissipated_priority=None  power_dissipated=uuberenndt W  power_dissipated_nominal_specify=off  power_dissipated_nominal_unit=W  power_dissipated_nominal_value=zxdbkerarj  thermal_network_parameterization=jgdhoyqkgb  Rth=zfnbvvzomp K/W  Rth_Foster=efezaqcttv K/W  thermal_mass_parameterization=dmbasvufig  thermal_mass=tokjdiqqfg J/K  thermal_mass_Foster=mahdpsfuip J/K  thermal_time_constant=zmmzrqwbmo s  thermal_time_constant_Foster=bacfszxpmj s  thermal_mass_initial_temperatures=jgpescfmbb degC
      settings: SourceProductName=Simscape Electrical  InternalSimscapePortConfiguration="{\"Bottom\":[],\"Left\":[{\"id\":\"p\",\"label\":\"\",\"type\":\"foundation.electrical.electrical\"},{\"id\":\"H\",\"label\":\"H\",\"type\":\"foundation.thermal.thermal\"}],\"Right\":[{\"id\":\"n\",\"label\":\"\",\"type\":\"foundation.electrical.electrical\"}],\"Top\":[]}"
  Redacted_467 : ee_lib/Semiconductors & Converters/Diode  ModelType=zwlyghrise  Vf=euzwuqecka V  Ron=sqqlvgrmjb Ohm  Goff=bmldewftqw S  prmExp=fjuhevddso  I12=yyjhzztotg A  V12=uojrvplvvj V  IS=cfmsrmnpsn A  ec=bhxifbozbf  I1=qnabjxlwpe A  V1=qvsekpkmcx V  RS=oaatpqtofx Ohm  Tmeas=fxzrhnbzxw degC  N_series=frjvnwrrls  N_parallel=umpwwncuya  Rz=boqmxjzfda Ohm  BV=vwgvvolkfz V  C_param=wwurieaact  CJ=mhbbjauuqe pF  CJ0=fihxqirexw pF  VJ=kwlcvjkmvx V  Mgrad=wmvcjduqzw  Vvec=eostyisdez V  Cvec=zqwmellhog pF  FC=aywdksybze  Q_param=xegpbnqmsp  iRM=thzcufmasx A  iF=jtqklphmoa A  didt=uaygsalief A/us  trr_factor=hauvgridjf  trr=msqoixcjlj ns  Qrr=tucpeotqzo s*uA  TT=fpdueotkxs ns  tau=uwhowgbepa ns  T_param=yukufyyeby  IS_T2=slesqmfvks A  I1_T2=cyohlfwokl A  V1_T2=zciacdqqef V  Tmeas2=odhefydsxa degC  EG_param=yjfkbklesn  EG=jqezgnscdw eV  XTI_param=etnksvgilo  XTI=pgrzlvrznx  dBVdT=thityipxbq V/K  Tdevice=aamobpecky degC  i_specify=off  i_priority=None  i=knehxtpuza A  i_nominal_specify=off  i_nominal_unit=A  i_nominal_value=tsfgfpsoce  v_specify=off  v_priority=None  v=ztgmiqkbgh V  v_nominal_specify=off  v_nominal_unit=V  v_nominal_value=npuzlaeycc  i_capacitor_specify=off  i_capacitor_priority=None  i_capacitor=tevzevklgo A  i_capacitor_nominal_specify=off  i_capacitor_nominal_unit=A  i_capacitor_nominal_value=ptrppgqifa  v_capacitor_specify=off  v_capacitor_priority=None  v_capacitor=mdzmhpiquf V  v_capacitor_nominal_specify=off  v_capacitor_nominal_unit=V  v_capacitor_nominal_value=dwuxzrnnxv  power_dissipated_specify=off  power_dissipated_priority=None  power_dissipated=maylsgmrfw W  power_dissipated_nominal_specify=off  power_dissipated_nominal_unit=W  power_dissipated_nominal_value=gjltmbkcbk  thermal_network_parameterization=ktvcgskyws  Rth=nrirmgsmli K/W  Rth_Foster=jwhpklzmjv K/W  thermal_mass_parameterization=ocwdrvizwl  thermal_mass=rzcsouwcda J/K  thermal_mass_Foster=ibedqwexgm J/K  thermal_time_constant=rszlxecmsr s  thermal_time_constant_Foster=vuiazerwrm s  thermal_mass_initial_temperatures=jaceaqhftk degC
      settings: SourceProductName=Simscape Electrical  InternalSimscapePortConfiguration="{\"Bottom\":[],\"Left\":[{\"id\":\"p\",\"label\":\"\",\"type\":\"foundation.electrical.electrical\"},{\"id\":\"H\",\"label\":\"H\",\"type\":\"foundation.thermal.thermal\"}],\"Right\":[{\"id\":\"n\",\"label\":\"\",\"type\":\"foundation.electrical.electrical\"}],\"Top\":[]}"
  Redacted_5096 : fl_lib/Electrical/Electrical Elements/Switch  R_closed=bhwptyrbvv Ohm  G_open=yibdhtabty 1/Ohm  Threshold=vyhtmbwtyb  i_specify=off  i_priority=None  i=emdqjvxpbx A  i_nominal_specify=off  i_nominal_unit=A  i_nominal_value=amqougtlub  v_specify=off  v_priority=None  v=txxyluqvej V  v_nominal_specify=off  v_nominal_unit=V  v_nominal_value=rdvslnaxld
      settings: SourceProductName=Simscape
  Redacted_8012 : fl_lib/Electrical/Electrical Elements/Switch  R_closed=anuzxeezmu Ohm  G_open=brgjbcwtyq 1/Ohm  Threshold=smlifqbzgv  i_specify=off  i_priority=None  i=ikjmsfyjtt A  i_nominal_specify=off  i_nominal_unit=A  i_nominal_value=jqmpassdoj  v_specify=off  v_priority=None  v=uwwbrmnmns V  v_nominal_specify=off  v_nominal_unit=V  v_nominal_value=gorbelvbmd
      settings: SourceProductName=Simscape
  Redacted_9794 : ee_lib/Passive/Thermal/Thermal Resistor  R=cmrcgyiplk K/W  T_specify=off  T_priority=None  T=fenyjgxqyv K  T_nominal_specify=off  T_nominal_unit=K  T_nominal_value=lgimuztorp  Q_specify=off  Q_priority=None  Q=ufcrfapicn W  Q_nominal_specify=off  Q_nominal_unit=W  Q_nominal_value=gfckcwtrdf
      settings: SourceProductName=Simscape Electrical  SourceProductBaseCode=PS  InternalSimscapePortConfiguration="{\"Bottom\":[],\"Left\":[{\"id\":\"A\",\"label\":\"A\",\"type\":\"foundation.thermal.thermal\"}],\"Right\":[{\"id\":\"B\",\"label\":\"B\",\"type\":\"foundation.thermal.thermal\"}],\"Top\":[]}"
  Redacted_9473 : PMIOPort  Side=Left
  Redacted_5887 : PMIOPort  Port=2  Side=Left
  Redacted_5665 : PMIOPort  Port=3  Side=Right
  Redacted_3172 : PMIOPort  Port=4  Side=Right
  Redacted_6215 : PMIOPort  Port=5  Side=Left
  Redacted_5523 : PMIOPort  Port=6  Side=Right
  connections:
  Redacted_24/LConn2 -- Redacted_1835/LConn1
  Redacted_2325/RConn1 -- Redacted_6215/RConn1
  Redacted_3172/RConn1 -- Redacted_5096/RConn2
  Redacted_8012/RConn1 -- Redacted_5096/RConn1 -- Redacted_5523/RConn1
  Redacted_9794/RConn1 -- Redacted_2325/LConn1 -- Redacted_1835/RConn1
  Redacted_9473/RConn1 -- Redacted_467/RConn1
  Redacted_467/LConn1 -- Redacted_8012/LConn1
  Redacted_5665/RConn1 -- Redacted_8012/RConn2
  Redacted_467/LConn2 -- Redacted_9794/LConn1
  Redacted_24/RConn1 -- Redacted_5096/LConn1
  Redacted_24/LConn1 -- Redacted_5887/RConn1
